simulink model "Simulink_model_Imbalances"  (R2025a)
settings: Solver=FixedStepAuto  StartTime=0.0  StopTime=3000  FixedStep=0.001  RelTol=1e-3
undefined symbols (not defined in the file or in its folder): Value
settings Model: Creator=AliRanjbar  LastModifiedBy=AliRanjbar

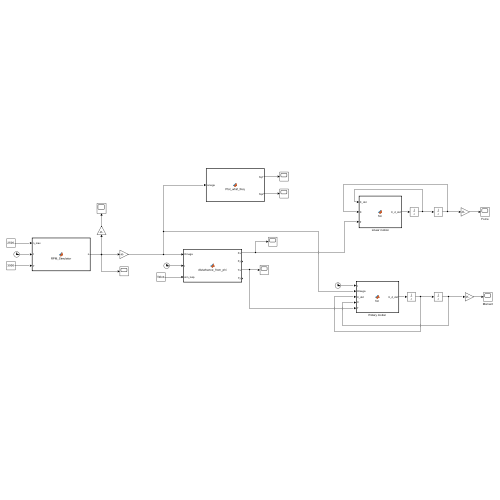
[thumbnail: Simulink's stored preview of the top-level diagram]
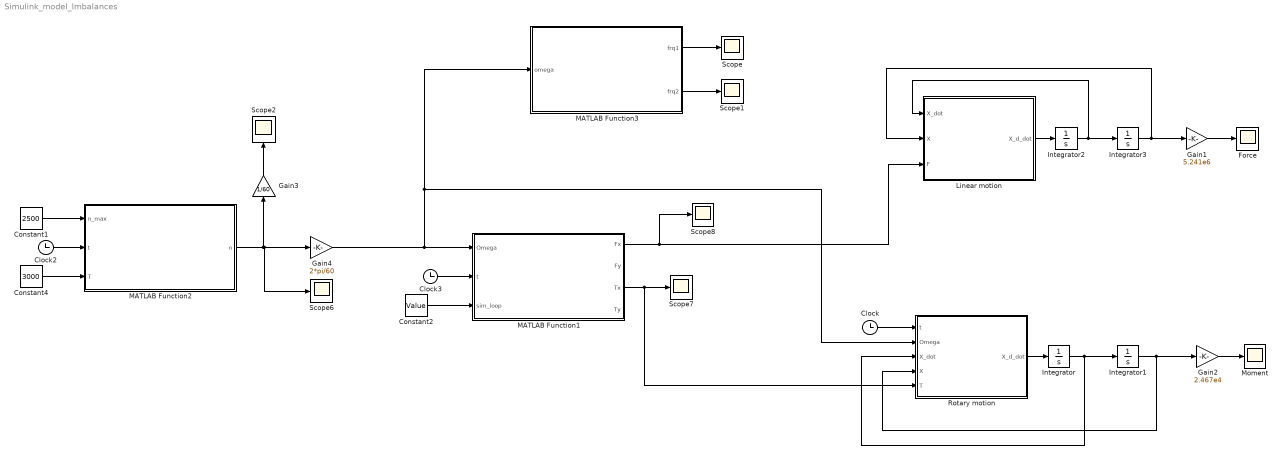
== system Simulink_model_Imbalances ==
  Clock : Clock
  Clock2 : Clock
  Clock3 : Clock
  Constant1 : Constant  Value=2500
  Constant2 : Constant  Value=Value
  Constant4 : Constant  Value=3000
  Force : Scope
      settings: ActiveDisplayYMinimum=-4.7921699002703129  ActiveDisplayYMaximum=4.7923767911849975  DataLoggingVariableName=Signal  DataLoggingSaveFormat=Structure
  Gain1 : Gain  Gain=5.241e6
  Gain2 : Gain  Gain=2.467e4
  Gain3 : Gain  Gain=1/60
  Gain4 : Gain  Gain=2*pi/60
  Integrator{,1..3} (4 alike) : Integrator  InitialCondition=[0 ;0]
  Linear motion : MATLAB Function  TreatAsAtomicUnit=on
  MATLAB Function1 : MATLAB Function  TreatAsAtomicUnit=on
  MATLAB Function2 : MATLAB Function  TreatAsAtomicUnit=on
  MATLAB Function3 : MATLAB Function  TreatAsAtomicUnit=on
  Moment : Scope
      settings: ActiveDisplayYMinimum=-2.8332131386682615  ActiveDisplayYMaximum=2.8331873339770586  DataLoggingVariableName=Moment  DataLoggingSaveFormat=Structure
  Rotary motion : MATLAB Function  TreatAsAtomicUnit=on
  Scope{,1..2,6..8} (6 alike) : Scope
      Scope settings: ActiveDisplayYMinimum=96.2246333874862  ActiveDisplayYMaximum=129.92118060739998  DataLoggingVariableName=WhirlF1  DataLoggingSaveFormat=Structure
      Scope1 settings: ActiveDisplayYMinimum=74.117609178828531  ActiveDisplayYMaximum=102.42503021288302  DataLoggingVariableName=WhirlF2  DataLoggingSaveFormat=Structure
      Scope2 settings: ActiveDisplayYMinimum=-5.2083333333333321  ActiveDisplayYMaximum=46.875  DataLoggingVariableName=RateofRotation  DataLoggingSaveFormat=Structure
      Scope6 settings: ActiveDisplayYMinimum=-1  ActiveDisplayYMaximum=1  DataLoggingVariableName=RPM_t  DataLoggingSaveFormat=Structure
      Scope7 settings: ActiveDisplayYMinimum=-1  ActiveDisplayYMaximum=1  DataLoggingVariableName=ScopeData7
      Scope8 settings: ActiveDisplayYMinimum=-0.98472898438343692  ActiveDisplayYMaximum=0.9842182198338838  DataLoggingVariableName=ScopeData8
  wires:
  Rotary motion/1(X_d_dot) -> Integrator/1
  Integrator/1 -> Rotary motion/3(X_dot), Integrator1/1
  Integrator1/1 -> Rotary motion/4(X), Gain2/1
  Clock/1 -> Rotary motion/1(t)
  Integrator3/1 -> Gain1/1, Linear motion/2(X)
  Integrator2/1 -> Integrator3/1, Linear motion/1(X_dot)
  Linear motion/1(X_d_dot) -> Integrator2/1
  Constant1/1 -> MATLAB Function2/1(n_max)
  Clock2/1 -> MATLAB Function2/2(t)
  Clock3/1 -> MATLAB Function1/2(t)
  MATLAB Function1/1(Fx) -> Linear motion/3(F), Scope8/1
  Constant4/1 -> MATLAB Function2/3(T)
  MATLAB Function1/3(Tx) -> Rotary motion/5(T), Scope7/1
  Gain1/1 -> Force/1
  MATLAB Function2/1(n) -> Gain4/1, Scope6/1, Gain3/1
  Gain2/1 -> Moment/1
  Constant2/1 -> MATLAB Function1/3(sim_loop)
  Gain4/1 -> Rotary motion/2(Omega), MATLAB Function3/1(omega), MATLAB Function1/1(Omega)
  MATLAB Function3/1(frq1) -> Scope/1
  MATLAB Function3/2(frq2) -> Scope1/1
  Gain3/1 -> Scope2/1

== matlab function Simulink_model_Imbalances/Linear motion ==
  data: X_dot input; X input; X_d_dot output; F input
function X_d_dot  = fcn(X_dot,X,F)
%% coefficients
Ct=200;
kt=5.241e6;
rd=.16;
rs=.16;
h=.048;
Us=.716e-5;%kgm
Ud=29.54e-7;%kgm2
Mw=5.9;

md=Ud/(2*rd*h);
ms=Us/rs;
Mt=Mw+ms+2*md;


%% Matrices
A=diag([Mt Mt]);
C=diag([Ct Ct]);
K=diag([kt kt]);

%% Dynamics
X_d_dot=inv(A)*(-(C*X_dot+K*X)+F);

== matlab function Simulink_model_Imbalances/Rotary motion ==
  data: t input; X_d_dot output; Omega input; X_dot input; X input; T input
function X_d_dot  = fcn(t,Omega,X_dot,X,T)
%% coefficients
Irr=.063;
Izz=.075;
Ct=.942;
kt=2.467e4;
rd=.16;
rs=.16;
h=.048;
Us=.716e-5;%kgm
Ud=29.54e-7;%kgm2

md=Ud/(2*rd*h);
ms=Us/rs;

It=2*md*rd^2+ms*rd^2;

%% Matrices
A=[Irr .5*It*sin(2*Omega*t); .5*It*sin(2*Omega*t) Irr];
B=[-It*sin(2*Omega*t) Izz; -Izz It*sin(2*Omega*t)];
C=diag([Ct Ct]);
K=diag([kt kt]);

%% Dynamics
X_d_dot=inv(A)*(-(Omega*B+C)*X_dot-K*X+T);

== matlab function Simulink_model_Imbalances/MATLAB Function3 ==
  settings: updateMethod=DISCRETE
  data: omega input; frq1 output; frq2 output

function [frq1, frq2]= Plot_whirl_freq(omega)

Irr=.063;
Izz=.075;
Ct=.942;
kt=2.467e4;
rd=.16;
rs=.16;
h=.048;
Us=.716e-5;%kgm
Ud=29.54e-7;%kgm2

md=Ud/(2*rd*h);
ms=Us/rs;

It=2*md*rd^2+ms*rd^2;

frq1=(omega*Izz/2/Irr+sqrt((omega*Izz/2/Izz)^2+(kt/Irr)))/2/pi;
frq2=(-omega*Izz/2/Irr+sqrt((omega*Izz/2/Izz)^2+(kt/Irr)))/2/pi;
end

== matlab function Simulink_model_Imbalances/MATLAB Function1 ==
  settings: updateMethod=DISCRETE
  data: Omega input; Fx output; Fy output; Tx output; Ty output; t input; sim_loop input
function [Fx, Fy, Tx, Ty] = disturbance_from_phi(Omega,t,sim_loop)

    h_f = [1.0000, 2.0000, 3.0000, 4.0000, 4.4300, 5.0000, 5.3800, 5.6000, 6.0000, 6.3900];
    C_f = [0.7852, 0.2984, 0.0777, 0.1036, 0.1280, 0.0849, 0.0985, 0.1849, 0.0618, 0.0402];

    h_t = [1.0000, 2.0000, 2.9000, 3.8800, 4.0000, 4.4300, 5.2000, 5.4000, 5.6000, 5.8100, 6.0000];
    C_t = [0.3239, 0.0744, 0.0309, 0.0472, 0.0121, 0.0412, 0.0924, 0.1027, 0.0630, 0.0851, 0.0173];



    % sim_loop=2;
    % h_f=h_f(sim_loop);
    % C_f=1e-7*((60/2/pi)^2)*C_f(sim_loop);
    % 
    % h_t=h_t(sim_loop);
    % C_t=1e-7*((60/2/pi)^2)*C_t(sim_loop);

    C_f_all = 1e-7 * (60/(2*pi))^2 .* C_f;
    C_t_all = 1e-7 * (60/(2*pi))^2 * C_t;

% % Sum all harmonics
    Fx = 0;  Fy = 0;
    Tx = 0;  Ty = 0;

% 
% 
%     % 
%     % % % Fx =-Us * Omega^2 * sin(Omega*t);
%     % % % Fy = Us * Omega^2 * cos(Omega*t);
%     % Fx = -C_f * Omega^2 * sin(h_f*Omega*t);
%     % Fy =  C_f * Omega^2 * cos(h_f*Omega*t);
% 
% 
    for i = 1:length(h_f)
        Fx = Fx - C_f_all(i)* Omega^2 * sin(h_f(i)*Omega*t);
        % Fy = Fy + C_f_all(i) * Omega^2 * cos(h_f(i)*Omega*t);
    end
% 
%     % 
%     % 
%     Tx = C_t * Omega^2 * cos(h_t.*Omega*t);
%     Ty = C_t * Omega^2 * sin(h_t.*Omega*t);

 
    for i = 1:length(h_t)
        Tx = Tx + C_t_all(i) * Omega^2 * cos(h_t(i)*Omega*t);
        % Ty = Ty + C_t_all(i) * Omega^2 * sin(h_t(i)*Omega*t);
    end



    
end

== matlab function Simulink_model_Imbalances/MATLAB Function2 ==
  settings: updateMethod=DISCRETE
  data: n_max input; n output; t input; T input
function n  = RPM_Simulator(n_max, t,T)

% Wheel speed [rpm]
if t <= T
    n = n_max * (t / T)^2;
else
    n = n_max;

end
